simulink library "lib_fuel_converter3"  (Simulink 4.1.1)
values from neighbouring files (symbols this model uses):
  logFlag = 1    [advSACompMaskInit.m]    (also in advSACompMaskInitR13.m)
undefined symbols (not defined in the file or in its folder): air_cp, amb_tmp, cyc_mph, ex_gas_cp, fc_acc_mass, fc_base_mass, fc_c2i_th_cond, fc_c_init_tmp, fc_cl2h_eff, fc_CO2_to_FUELgps, fc_cold, fc_cold_tmp, fc_cp, fc_ct_trq, fc_emisv, fc_ext_sarea, fc_fuel_den, fc_fuel_lhv, fc_h2x_th_cond, fc_h_air_flow, fc_h_cp, fc_h_init_tmp, fc_hood_emisv, fc_hood_sarea, fc_i2x_th_cond, fc_i_init_tmp, fc_inertia, fc_map_spd, fc_map_trq, fc_max_trq, fc_nn_model_name, fc_pwr_scale, fc_spd_scale, fc_trq_scale, fc_tstat, fc_x_init_tmp, fd_ratio, gb_num_init, gb_ratio, generalName, pow, vc_idle_bool, vc_idle_spd, vc_key_on, veh_glider_mass, wh_radius
libraries: lib_fuel_converter3 x4, lib_etc x4, lib_fuel_converter x2, lib_fuel_converter2 x1
(part 2 of 9)

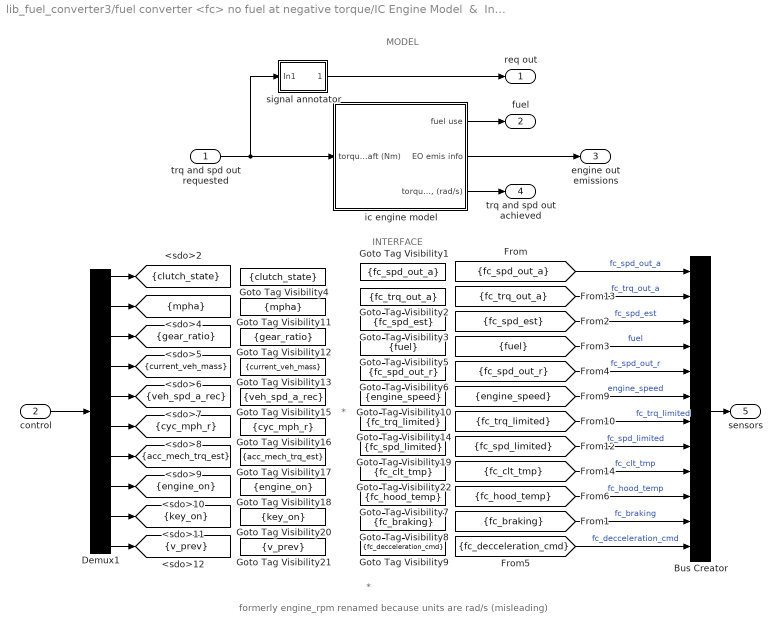
== system lib_fuel_converter3/fuel converter <fc> no fuel at negative torque/IC Engine Model  &  Interface ==
  note: *
  note: *
  note: formerly
      | engine_rpm
      | renamed because
      | units are rad/s
      |  (misleading)
  note: MODEL
  note: INTERFACE
  trq and spd out requested : Inport  Port=1  LatchInput=off
  control : Inport  Port=2  LatchInput=off
  Bus Creator : BusCreator  Inputs=12
  Demux1 : Demux  Outputs=10  BusSelectionMode=off
  Goto Tag Visibility1 : GotoTagVisibility  GotoTag=fc_spd_out_a
  Goto Tag Visibility10 : GotoTagVisibility  GotoTag=engine_speed
  Goto Tag Visibility11 : GotoTagVisibility  GotoTag=mpha
  Goto Tag Visibility12 : GotoTagVisibility  GotoTag=gear_ratio
  Goto Tag Visibility13 : GotoTagVisibility  GotoTag=current_veh_mass
  Goto Tag Visibility14 : GotoTagVisibility  GotoTag=fc_trq_limited
  Goto Tag Visibility15 : GotoTagVisibility  GotoTag=veh_spd_a_rec
  Goto Tag Visibility16 : GotoTagVisibility  GotoTag=cyc_mph_r
  Goto Tag Visibility17 : GotoTagVisibility  GotoTag=acc_mech_trq_est
  Goto Tag Visibility18 : GotoTagVisibility  GotoTag=engine_on
  Goto Tag Visibility19 : GotoTagVisibility  GotoTag=fc_spd_limited
  Goto Tag Visibility2 : GotoTagVisibility  GotoTag=fc_trq_out_a
  Goto Tag Visibility20 : GotoTagVisibility  GotoTag=key_on
  Goto Tag Visibility21 : GotoTagVisibility  GotoTag=v_prev
  Goto Tag Visibility22 : GotoTagVisibility  GotoTag=fc_clt_tmp
  Goto Tag Visibility3 : GotoTagVisibility  GotoTag=fc_spd_est
  Goto Tag Visibility4 : GotoTagVisibility  GotoTag=clutch_state
  Goto Tag Visibility5 : GotoTagVisibility  GotoTag=fuel
  Goto Tag Visibility6 : GotoTagVisibility  GotoTag=fc_spd_out_r
  Goto Tag Visibility7 : GotoTagVisibility  GotoTag=fc_hood_temp
  Goto Tag Visibility8 : GotoTagVisibility  GotoTag=fc_braking
  Goto Tag Visibility9 : GotoTagVisibility  GotoTag=fc_decceleration_cmd
  ic engine model : Subsystem
      settings: RTWFcnNameOpts=Auto  RTWFileNameOpts=Auto
  signal annotator : Subsystem
      settings: RTWFcnNameOpts=Auto  RTWFileNameOpts=Auto
  req out : Outport  Port=1
  fuel : Outport  Port=2
  engine out emissions : Outport  Port=3
  trq and spd out achieved : Outport  Port=4
  sensors : Outport  Port=5
  tag scope: acc_mech_trq_est=scoped, clutch_state=scoped, current_veh_mass=scoped, cyc_mph_r=scoped, engine_on=scoped, gear_ratio=scoped, key_on=scoped, mpha=scoped, v_prev=scoped, veh_spd_a_rec=scoped
  wires:
  [fc_decceleration_cmd] -> Bus Creator/12  "fc_decceleration_cmd"
  Demux1/1 -> [clutch_state]
  Demux1/2 -> [mpha]
  Demux1/3 -> [gear_ratio]
  Demux1/4 -> [current_veh_mass]
  Demux1/5 -> [veh_spd_a_rec]
  Demux1/6 -> [cyc_mph_r]
  Demux1/7 -> [acc_mech_trq_est]
  Demux1/8 -> [engine_on]
  Demux1/9 -> [key_on]
  Demux1/10 -> [v_prev]
  [fc_spd_out_a] -> Bus Creator/1  "fc_spd_out_a"
  [fc_trq_out_a] -> Bus Creator/2  "fc_trq_out_a"
  [fc_spd_est] -> Bus Creator/3  "fc_spd_est"
  [fuel] -> Bus Creator/4  "fuel"
  [fc_spd_out_r] -> Bus Creator/5  "fc_spd_out_r"
  [engine_speed] -> Bus Creator/6  "engine_speed"
  [fc_trq_limited] -> Bus Creator/7  "fc_trq_limited"
  [fc_spd_limited] -> Bus Creator/8  "fc_spd_limited"
  [fc_clt_tmp] -> Bus Creator/9  "fc_clt_tmp"
  [fc_hood_temp] -> Bus Creator/10  "fc_hood_temp"
  trq and spd out requested/1 -> ic engine model/1(torque and speed  req'd at engine  output shaft (Nm)), signal annotator/1(In1)
  ic engine model/1(fuel use) -> fuel/1
  ic engine model/2(EO emis info) -> engine out emissions/1
  ic engine model/3("torque and speed  avail. to driveline (Nm), (rad/s)") -> trq and spd out achieved/1
  control/1 -> Demux1/1
  Bus Creator/1 -> sensors/1
  signal annotator/1(Out1) -> req out/1
  [fc_braking] -> Bus Creator/11  "fc_braking"

== system lib_fuel_converter3/fuel converter <fc> no fuel at negative torque/help ==

== system lib_fuel_converter3/Fuel Converter Control/Fuel Converter Control conventional ic engine/conventional IC engine ==
  note: Controls for Fuel Converter:
      | IC Engine
  Bus Creator : BusCreator  Inputs=10
  Bus Selector1 : BusSelector  OutputSignals=clutch_state  MuxedOutput=off
  Bus Selector2 : BusSelector  OutputSignals=shifting  MuxedOutput=off
  Bus Selector3 : BusSelector  OutputSignals=acc_mech_pwr_a  MuxedOutput=off
  Bus Selector4 : BusSelector  OutputSignals=v_prev  MuxedOutput=off
  Bus Selector5 : BusSelector  OutputSignals=cycle_mph_r  MuxedOutput=off
  Bus Selector6 : BusSelector  OutputSignals=veh_spd_a_rec  MuxedOutput=off
  Bus Selector7 : BusSelector  OutputSignals=gear_ratio  MuxedOutput=off
  Bus Selector8 : BusSelector  OutputSignals=current_veh_mass  MuxedOutput=off
  Bus Selector9 : BusSelector  OutputSignals=mpha  MuxedOutput=off
  Fuel Converter Control : Subsystem
      settings: RTWFcnNameOpts=Auto  RTWFileNameOpts=Auto
  Memory{1..3,5} (4 alike) : Memory  X0=0  InheritSampleTime=off
      settings: RTWStateStorageClass=Auto
  tag scope: fcControl=global
  wires:
  Bus Selector2/1 -> Fuel Converter Control/9(shifting)  "<shifting>"
  Bus Selector7/1 -> Fuel Converter Control/3(gear_ratio)  "<gear_ratio>"
  Bus Selector1/1 -> Fuel Converter Control/1(clutch_state)  "<clutch_state>"
  [clControl] -> Bus Selector1/1
  [gbControl] -> Bus Selector7/1
  [fcSensors] -> Fuel Converter Control/8(fcSensors)
  [vehReqOut] -> Bus Selector4/1
  Bus Selector4/1 -> Fuel Converter Control/10(v_prev)  "<v_prev>"
  [gbControl] -> Bus Selector2/1
  [accSensors] -> Bus Selector3/1
  Bus Selector3/1 -> Memory5/1  "<acc_mech_pwr_a>"
  Memory5/1 -> Fuel Converter Control/7(acc_mech_trq_est)
  [cycReqOut] -> Bus Selector5/1
  Bus Selector5/1 -> Memory3/1  "<cycle_mph_r>"
  [vehSensors] -> Bus Selector6/1
  Bus Selector6/1 -> Memory2/1  "<veh_spd_a_rec>"
  [cycSensors] -> Bus Selector8/1
  Bus Selector8/1 -> Fuel Converter Control/4(current_veh_mass)  "<current_veh_mass>"
  [vehSensors] -> Bus Selector9/1
  Bus Selector9/1 -> Memory1/1  "<mpha>"
  Fuel Converter Control/10(v_prev out) -> Bus Creator/10  "v_prev"
  Fuel Converter Control/9(key_on out) -> Bus Creator/9  "key_on"
  Fuel Converter Control/8(engine_on out) -> Bus Creator/8  "engine_on"
  Fuel Converter Control/7(acc_mech_trq_est out) -> Bus Creator/7  "acc_mech_trq_est"
  Fuel Converter Control/6(cyc_mph_r out) -> Bus Creator/6  "cyc_mph_r_prev"
  Fuel Converter Control/5(veh spd a rec out) -> Bus Creator/5  "veh_spd_a_rec_prev"
  Fuel Converter Control/4(current veh mass out) -> Bus Creator/4  "current_veh_mass"
  Fuel Converter Control/3(gear_ratio out) -> Bus Creator/3  "gear_ratio"
  Fuel Converter Control/2(miles per hour out) -> Bus Creator/2  "mpha_prev"
  Fuel Converter Control/1(clutch state out) -> Bus Creator/1  "clutch_state"
  Bus Creator/1 -> [fcControl]
  Memory1/1 -> Fuel Converter Control/2(mpha(t-1) (prev))
  Memory2/1 -> Fuel Converter Control/5(veh_spd_a_rec(t-1) (prev))
  Memory3/1 -> Fuel Converter Control/6(cyc_mph_r(t-1) (prev))

== system lib_fuel_converter3/configurable subsystems/fuel use and EO emis/Block NOTES ==
  note: This block determines actual fuel use and engine-out emissions
      | given the fully hot values and the engine coolant temperature.
      | The correlations used here were developed at NREL using
      | FTP data collected under subcontract by JDM & Associates.
      | Note: PM hot/cold relation assumed same as HC

== system lib_fuel_converter3/configurable subsystems/fuel use and EO emis/HOT engine maps ==
  T (Nm) : Inport  Port=1  LatchInput=off
  w (rad/s) : Inport  Port=2  LatchInput=off
  Enable : EnablePort  StatesWhenEnabling=reset
  Block NOTES : Subsystem
      settings: RTWFcnNameOpts=Auto  RTWFileNameOpts=Auto
      mask Display: disp('Block\nNOTES')
  CO (g/s) : Subsystem  mask(2-D Table Lookup){@1=fc_map_spd*fc_spd_scale, @2=fc_map_trq*fc_trq_scale, @3=fc_co_map*fc_spd_scale*fc_trq_scale}
      mask prompts: @1 "X Index"; @2 "Y Index"; @3 "Table"
      mask help:
      | Two Dimensional Table Lookup
      | The first input corresponds to X Index and the second input corresponds to the Y Index
      mask init:
      | xindex=@1; yindex=@2; table=@3; sftab2chk(xindex,yindex,table);
      settings: RTWFcnNameOpts=Auto  RTWFileNameOpts=Auto
      mask Help: This block returns a linearly interpolated intersection from the table using the X index (which corresponds to the rows of the table) and the Y index (which corresponds to the columns of the table).  Extrapolation is used.
      mask Display: plot(-10,-10,110,110,[90,50,10],[90,40,30],[90,50,10],[50,26,20],[90,50,10],[22,13,10])
  Fcn3 : Fcn  Expr=(u(1)/1000)*ex_gas_cp*(u(2) - amb_tmp)
  HC (g/s) : Subsystem  mask(2-D Table Lookup){@1=fc_map_spd*fc_spd_scale, @2=fc_map_trq*fc_trq_scale, @3=fc_hc_map*fc_spd_scale*fc_trq_scale}
      mask prompts: @1 "X Index"; @2 "Y Index"; @3 "Table"
      mask help:
      | Two Dimensional Table Lookup
      | The first input corresponds to X Index and the second input corresponds to the Y Index
      mask init:
      | xindex=@1; yindex=@2; table=@3; sftab2chk(xindex,yindex,table);
      settings: RTWFcnNameOpts=Auto  RTWFileNameOpts=Auto
      mask Help: This block returns a linearly interpolated intersection from the table using the X index (which corresponds to the rows of the table) and the Y index (which corresponds to the columns of the table).  Extrapolation is used.
      mask Display: plot(-10,-10,110,110,[90,50,10],[90,40,30],[90,50,10],[50,26,20],[90,50,10],[22,13,10])
  MF,ex (g/s) : Subsystem  mask(2-D Table Lookup){@1=fc_map_spd*fc_spd_scale, @2=fc_map_trq*fc_trq_scale, @3=fc_exflow_map*fc_spd_scale*fc_trq_scale}
      mask prompts: @1 "X Index"; @2 "Y Index"; @3 "Table"
      mask help:
      | Two Dimensional Table Lookup
      | The first input corresponds to X Index and the second input corresponds to the Y Index
      mask init:
      | xindex=@1; yindex=@2; table=@3; sftab2chk(xindex,yindex,table);
      settings: RTWFcnNameOpts=Auto  RTWFileNameOpts=Auto
      mask Help: This block returns a linearly interpolated intersection from the table using the X index (which corresponds to the rows of the table) and the Y index (which corresponds to the columns of the table).  Extrapolation is used.
      mask Display: plot(-10,-10,110,110,[90,50,10],[90,40,30],[90,50,10],[50,26,20],[90,50,10],[22,13,10])
  MinMax : MinMax  Function=min  Inputs=2
  Mux : Mux  Inputs=4
      settings: DisplayOption=none
  Mux4 : Mux  Inputs=2
      settings: DisplayOption=none
  NOx (g/s) : Subsystem  mask(2-D Table Lookup){@1=fc_map_spd*fc_spd_scale, @2=fc_map_trq*fc_trq_scale, @3=fc_nox_map*fc_spd_scale*fc_trq_scale}
      mask prompts: @1 "X Index"; @2 "Y Index"; @3 "Table"
      mask help:
      | Two Dimensional Table Lookup
      | The first input corresponds to X Index and the second input corresponds to the Y Index
      mask init:
      | xindex=@1; yindex=@2; table=@3; sftab2chk(xindex,yindex,table);
      settings: RTWFcnNameOpts=Auto  RTWFileNameOpts=Auto
      mask Help: This block returns a linearly interpolated intersection from the table using the X index (which corresponds to the rows of the table) and the Y index (which corresponds to the columns of the table).  Extrapolation is used.
      mask Display: plot(-10,-10,110,110,[90,50,10],[90,40,30],[90,50,10],[50,26,20],[90,50,10],[22,13,10])
  O2 (g/s) : Subsystem  mask(2-D Table Lookup){@1=fc_map_spd*fc_spd_scale, @2=fc_map_trq*fc_trq_scale, @3=fc_o2_map*fc_spd_scale*fc_trq_scale}
      mask prompts: @1 "X Index"; @2 "Y Index"; @3 "Table"
      mask help:
      | Two Dimensional Table Lookup
      | The first input corresponds to X Index and the second input corresponds to the Y Index
      mask init:
      | xindex=@1; yindex=@2; table=@3; sftab2chk(xindex,yindex,table);
      settings: RTWFcnNameOpts=Auto  RTWFileNameOpts=Auto
      mask Help: This block returns a linearly interpolated intersection from the table using the X index (which corresponds to the rows of the table) and the Y index (which corresponds to the columns of the table).  Extrapolation is used.
      mask Display: plot(-10,-10,110,110,[90,50,10],[90,40,30],[90,50,10],[50,26,20],[90,50,10],[22,13,10])
  PM (g/s) : Subsystem  mask(2-D Table Lookup){@1=fc_map_spd*fc_spd_scale, @2=fc_map_trq*fc_trq_scale, @3=fc_pm_map*fc_spd_scale*fc_trq_scale}
      mask prompts: @1 "X Index"; @2 "Y Index"; @3 "Table"
      mask help:
      | Two Dimensional Table Lookup
      | The first input corresponds to X Index and the second input corresponds to the Y Index
      mask init:
      | xindex=@1; yindex=@2; table=@3; sftab2chk(xindex,yindex,table);
      settings: RTWFcnNameOpts=Auto  RTWFileNameOpts=Auto
      mask Help: This block returns a linearly interpolated intersection from the table using the X index (which corresponds to the rows of the table) and the Y index (which corresponds to the columns of the table).  Extrapolation is used.
      mask Display: plot(-10,-10,110,110,[90,50,10],[90,40,30],[90,50,10],[50,26,20],[90,50,10],[22,13,10])
  Product : Product  Inputs=2  Multiplication=Element-wise(.*)  SaturateOnIntegerOverflow=on
  Saturation : Saturate  UpperLimit=max(fc_map_trq*fc_trq_scale)  LowerLimit=min(fc_map_trq*fc_trq_scale)  LinearizeAsGain=on
  Saturation1 : Saturate  UpperLimit=max(fc_map_spd*fc_spd_scale)  LowerLimit=min(fc_map_spd*fc_spd_scale)  LinearizeAsGain=on
  Sum5 : Sum  Inputs=-+  SaturateOnIntegerOverflow=on
  Sum6 : Sum  Inputs=-+  SaturateOnIntegerOverflow=on
  Tex,eo (C) : Subsystem  mask(2-D Table Lookup){@1=fc_map_spd*fc_spd_scale, @2=fc_map_trq*fc_trq_scale, @3=fc_extmp_map}
      mask prompts: @1 "X Index"; @2 "Y Index"; @3 "Table"
      mask help:
      | Two Dimensional Table Lookup
      | The first input corresponds to X Index and the second input corresponds to the Y Index
      mask init:
      | xindex=@1; yindex=@2; table=@3; sftab2chk(xindex,yindex,table);
      settings: RTWFcnNameOpts=Auto  RTWFileNameOpts=Auto
      mask Help: This block returns a linearly interpolated intersection from the table using the X index (which corresponds to the rows of the table) and the Y index (which corresponds to the columns of the table).  Extrapolation is used.
      mask Display: plot(-10,-10,110,110,[90,50,10],[90,40,30],[90,50,10],[50,26,20],[90,50,10],[22,13,10])
  fuel (g/s) : Subsystem  mask(2-D Table Lookup){@1=fc_map_spd*fc_spd_scale, @2=fc_map_trq*fc_trq_scale, @3=fc_fuel_map*fc_spd_scale*fc_trq_scale}
      mask prompts: @1 "X Index"; @2 "Y Index"; @3 "Table"
      mask help:
      | Two Dimensional Table Lookup
      | The first input corresponds to X Index and the second input corresponds to the Y Index
      mask init:
      | xindex=@1; yindex=@2; table=@3; sftab2chk(xindex,yindex,table);
      settings: RTWFcnNameOpts=Auto  RTWFileNameOpts=Auto
      mask Help: This block returns a linearly interpolated intersection from the table using the X index (which corresponds to the rows of the table) and the Y index (which corresponds to the columns of the table).  Extrapolation is used.
      mask Display: plot(-10,-10,110,110,[90,50,10],[90,40,30],[90,50,10],[50,26,20],[90,50,10],[22,13,10])
  lhv : Gain  Gain=fc_fuel_lhv  Multiplication=Element-wise(K.*u)  SaturateOnIntegerOverflow=on
  fc heat (W) : Outport  Port=1  OutputWhenDisabled=reset  InitialOutput=eps
  HOT fuel use (g/s) : Outport  Port=2  OutputWhenDisabled=reset  InitialOutput=eps
  HOT emis (g/s) : Outport  Port=3  OutputWhenDisabled=reset  InitialOutput=eps
  Ex Gas Flow (g/s) : Outport  Port=4  OutputWhenDisabled=reset  InitialOutput=eps
  Ex Gas Temp (C) : Outport  Port=5  OutputWhenDisabled=reset  InitialOutput=amb_tmp
  O2 exhaust (g/s) : Outport  Port=6  OutputWhenDisabled=reset  InitialOutput=0
  ex heat (W) : Outport  Port=7  OutputWhenDisabled=reset  InitialOutput=eps
  wires:
  PM (g/s)/1(table out) -> Mux/4
  HC (g/s)/1(table out) -> Mux/1
  CO (g/s)/1(table out) -> Mux/2
  NOx (g/s)/1(table out) -> Mux/3
  Mux/1 -> HOT emis (g/s)/1
  MF,ex (g/s)/1(table out) -> Ex Gas Flow (g/s)/1, Mux4/1
  Tex,eo (C)/1(table out) -> Ex Gas Temp (C)/1, Mux4/2
  Saturation1/1 -> NOx (g/s)/1(x0), MF,ex (g/s)/1(x0), Tex,eo (C)/1(x0), fuel (g/s)/1(x0), O2 (g/s)/1(x0), PM (g/s)/1(x0), CO (g/s)/1(x0), HC (g/s)/1(x0)
  Saturation/1 -> CO (g/s)/2(y0), MF,ex (g/s)/2(y0), Tex,eo (C)/2(y0), fuel (g/s)/2(y0), O2 (g/s)/2(y0), PM (g/s)/2(y0), NOx (g/s)/2(y0), HC (g/s)/2(y0)
  T (Nm)/1 -> Saturation/1, Product/1
  w (rad/s)/1 -> Saturation1/1, Product/2
  Mux4/1 -> Fcn3/1
  Sum5/1 -> fc heat (W)/1
  Fcn3/1 -> MinMax/1
  MinMax/1 -> Sum5/1, ex heat (W)/1
  Sum6/1 -> Sum5/2, MinMax/2
  Product/1 -> Sum6/1
  fuel (g/s)/1(table out) -> HOT fuel use (g/s)/1, lhv/1
  lhv/1 -> Sum6/2
  O2 (g/s)/1(table out) -> O2 exhaust (g/s)/1

== system lib_fuel_converter3/configurable subsystems/fuel use and EO emis/enhancedToWorkspace1 ==
  In1 : Inport  Port=1  LatchInput=off
  Terminator : Terminator
  wires:
  In1/1 -> Terminator/1

== system lib_fuel_converter3/configurable subsystems/fuel use and EO emis/enhancedToWorkspace10 ==
  In1 : Inport  Port=1  LatchInput=off
  Terminator : Terminator
  wires:
  In1/1 -> Terminator/1

== system lib_fuel_converter3/configurable subsystems/fuel use and EO emis/enhancedToWorkspace11 ==
  In1 : Inport  Port=1  LatchInput=off
  Terminator : Terminator
  wires:
  In1/1 -> Terminator/1

== system lib_fuel_converter3/configurable subsystems/fuel use and EO emis/enhancedToWorkspace12 ==
  In1 : Inport  Port=1  LatchInput=off
  Terminator : Terminator
  wires:
  In1/1 -> Terminator/1

== system lib_fuel_converter3/configurable subsystems/fuel use and EO emis/enhancedToWorkspace2 ==
  In1 : Inport  Port=1  LatchInput=off
  Terminator : Terminator
  wires:
  In1/1 -> Terminator/1

== system lib_fuel_converter3/configurable subsystems/fuel use and EO emis/enhancedToWorkspace3 ==
  In1 : Inport  Port=1  LatchInput=off
  Terminator : Terminator
  wires:
  In1/1 -> Terminator/1

== system lib_fuel_converter3/configurable subsystems/fuel use and EO emis/enhancedToWorkspace5 ==
  In1 : Inport  Port=1  LatchInput=off
  Terminator : Terminator
  wires:
  In1/1 -> Terminator/1

== system lib_fuel_converter3/configurable subsystems/fuel use and EO emis/enhancedToWorkspace6 ==
  In1 : Inport  Port=1  LatchInput=off
  Terminator : Terminator
  wires:
  In1/1 -> Terminator/1

== system lib_fuel_converter3/configurable subsystems/fuel use and EO emis/enhancedToWorkspace7 ==
  In1 : Inport  Port=1  LatchInput=off
  Terminator : Terminator
  wires:
  In1/1 -> Terminator/1

== system lib_fuel_converter3/configurable subsystems/fuel use and EO emis/enhancedToWorkspace8 ==
  In1 : Inport  Port=1  LatchInput=off
  Terminator : Terminator
  wires:
  In1/1 -> Terminator/1

== system lib_fuel_converter3/configurable subsystems/fuel use and EO emis/enhancedToWorkspace9 ==
  In1 : Inport  Port=1  LatchInput=off
  Terminator : Terminator
  wires:
  In1/1 -> Terminator/1

== system lib_fuel_converter3/configurable subsystems/fuel use and EO emis/fc temp ==
  note: h
  note: x
  note: i
  note: c
  veh spd (m/s) : Inport  Port=1  LatchInput=off
  key ON? : Inport  Orientation=down  Port=2  LatchInput=off
  fc ON? : Inport  Port=3  LatchInput=off
  Qfc (W) : Inport  Port=4  LatchInput=off
  1/ : Gain  Gain=1/(0.2*fc_base_mass*fc_pwr_scale*fc_cp)  Multiplication=Element-wise(K.*u)  SaturateOnIntegerOverflow=on
  1/Ci : Gain  Gain=1/(0.8*fc_base_mass*fc_pwr_scale*fc_cp)  Multiplication=Element-wise(K.*u)  SaturateOnIntegerOverflow=on
  1/Cx : Gain  Gain=1/(fc_acc_mass*fc_pwr_scale*fc_cp)  Multiplication=Element-wise(K.*u)  SaturateOnIntegerOverflow=on
  1/mcp : Gain  Gain=1/(0.1*veh_glider_mass*fc_pwr_scale*fc_h_cp)  Multiplication=Element-wise(K.*u)  SaturateOnIntegerOverflow=on
  Block NOTES : Subsystem
      settings: RTWFcnNameOpts=Auto  RTWFileNameOpts=Auto
      mask Display: disp('Block\nNOTES')
  Memory : Memory  X0=fc_h_init_tmp  InheritSampleTime=off
      settings: RTWStateStorageClass=Auto
  Mux3 : Mux  Inputs=4
      settings: DisplayOption=none
  Mux4 : Mux  Inputs=2
      settings: DisplayOption=none
  Qc : Sum  Inputs=++  SaturateOnIntegerOverflow=on
  Qc1 : Sum  Inputs=--+  SaturateOnIntegerOverflow=on
  Tcm : Integrator  ExternalReset=none  InitialConditionSource=internal  InitialCondition=fc_c_init_tmp  LimitOutput=off  UpperSaturationLimit=inf  LowerSaturationLimit=-inf  ShowSaturationPort=off  ShowStatePort=off  AbsoluteTolerance=auto
  Tcx : Integrator  ExternalReset=none  InitialConditionSource=internal  InitialCondition=fc_x_init_tmp  LimitOutput=off  UpperSaturationLimit=inf  LowerSaturationLimit=-inf  ShowSaturationPort=off  ShowStatePort=off  AbsoluteTolerance=auto
  Tcx1 : Integrator  ExternalReset=none  InitialConditionSource=internal  InitialCondition=fc_i_init_tmp  LimitOutput=off  UpperSaturationLimit=inf  LowerSaturationLimit=-inf  ShowSaturationPort=off  ShowStatePort=off  AbsoluteTolerance=auto
  Tm : Integrator  ExternalReset=none  InitialConditionSource=internal  InitialCondition=fc_h_init_tmp  LimitOutput=off  UpperSaturationLimit=inf  LowerSaturationLimit=-inf  ShowSaturationPort=off  ShowStatePort=off  AbsoluteTolerance=auto
  fc coolant : Subsystem  TreatAsAtomicUnit=on
      settings: RTWFcnNameOpts=Auto  RTWFileNameOpts=Auto
  fc mass heat flow : Subsystem
      settings: RTWFcnNameOpts=Auto  RTWFileNameOpts=Auto
  old fc coolant  temp. (C) : Subsystem
      settings: RTWFcnNameOpts=Auto  RTWFileNameOpts=Auto
  Tfc_old  (C) : Outport  Port=1  InitialOutput=0
  Qfc r,h : Outport  Port=2  InitialOutput=0
  Tfc  (C) : Outport  Port=3  InitialOutput=0
  tag scope: fc_hood_temp=scoped
  wires:
  Qc/1 -> 1//1
  1//1 -> Tcm/1
  Qfc (W)/1 -> Qc/1
  fc mass heat flow/1(Qfc_c) -> Qc/2
  Qc1/1 -> 1/Ci/1
  1/Ci/1 -> Tcx1/1
  Tcm/1 -> Mux3/1
  fc mass heat flow/2(Qfc_i) -> Qc1/3, fc coolant/2("Qfc_i ")
  fc coolant/2(Qfc_htr) -> Qc1/2, Mux4/2
  fc coolant/1(Qfc_rad) -> Qc1/1, Mux4/1
  Tcx1/1 -> fc coolant/1(Tcl), Mux3/2
  Mux4/1 -> Qfc r,h/1
  1/Cx/1 -> Tcx/1
  fc mass heat flow/3(Qfc_x) -> 1/Cx/1
  key ON?/1 -> fc coolant/Enable
  Tcx/1 -> Mux3/3
  Tm/1 -> Mux3/4, Memory/1
  1/mcp/1 -> Tm/1
  fc mass heat flow/4(Qfc_h) -> 1/mcp/1
  Mux3/1 -> fc mass heat flow/2(fc_temp), Tfc  (C)/1
  old fc coolant  temp. (C)/1(fc coolant  temp (C)) -> Tfc_old  (C)/1
  veh spd (m/s)/1 -> old fc coolant  temp. (C)/2(veh spd), fc mass heat flow/1(veh spd)
  fc ON?/1 -> old fc coolant  temp. (C)/1(fc on?)
  Memory/1 -> [fc_hood_temp]

== system lib_fuel_converter3/configurable subsystems/fuel use and EO emis/fc temp correct ==
  Coolant T (C) : Inport  Port=1  LatchInput=off
  HOT fuel use (g/s) : Inport  Port=2  LatchInput=off
  HOT emis (g/s) : Inport  Port=3  LatchInput=off
  T (Nm) : Inport  Port=4  LatchInput=off
  w (rad/s) : Inport  Port=5  LatchInput=off
  Enable : EnablePort  StatesWhenEnabling=reset
  =1: use map based =0: use constant equation based : Constant  Value=fc_cold
  Switch : Switch  Threshold=eps
  Switch1 : Switch  Threshold=eps
  fc temp correct Constant Correction Factors (Equation Based) : Subsystem  TreatAsAtomicUnit=on
      settings: RTWFcnNameOpts=Auto  RTWFileNameOpts=Auto
  fc temp correct Variable Correction Factors (Map Based) : Subsystem  TreatAsAtomicUnit=on
      settings: RTWFcnNameOpts=Auto  RTWFileNameOpts=Auto
  fc_cold=0 : Logic  Operator=NOT  Inputs=2
  fuel use (g/s) : Outport  Port=1  OutputWhenDisabled=reset  InitialOutput=0
  EO emis (g/s) : Outport  Port=2  OutputWhenDisabled=reset  InitialOutput=0
  wires:
  =1: use map based =0: use constant equation based/1 -> fc_cold=0/1, fc temp correct Variable Correction Factors (Map Based)/Enable
  Coolant T (C)/1 -> fc temp correct Constant Correction Factors (Equation Based)/1(Coolant T (C)), fc temp correct Variable Correction Factors (Map Based)/1(Coolant T (C))
  HOT fuel use (g/s)/1 -> fc temp correct Constant Correction Factors (Equation Based)/2(HOT fuel use (g/s)), fc temp correct Variable Correction Factors (Map Based)/2(HOT fuel use (g/s))
  HOT emis (g/s)/1 -> fc temp correct Constant Correction Factors (Equation Based)/3(HOT emis (g/s)), fc temp correct Variable Correction Factors (Map Based)/3(HOT emis (g/s))
  fc temp correct Constant Correction Factors (Equation Based)/1(fuel use (g/s)) -> Switch/1
  fc_cold=0/1 -> fc temp correct Constant Correction Factors (Equation Based)/Enable, Switch/2, Switch1/2
  fc temp correct Variable Correction Factors (Map Based)/1(fuel use (g/s)) -> Switch/3
  fc temp correct Constant Correction Factors (Equation Based)/2(EO emis (g/s)) -> Switch1/1
  fc temp correct Variable Correction Factors (Map Based)/2(EO emis (g/s)) -> Switch1/3
  Switch/1 -> fuel use (g/s)/1
  Switch1/1 -> EO emis (g/s)/1
  T (Nm)/1 -> fc temp correct Variable Correction Factors (Map Based)/4(T (Nm))
  w (rad/s)/1 -> fc temp correct Variable Correction Factors (Map Based)/5(w (rad/s))

== system lib_fuel_converter3/configurable subsystems/fuel use and EO emis Neural Network Model/HOT engine maps ==
  T (Nm) : Inport  Port=1  LatchInput=off
  w (rad/s) : Inport  Port=2  LatchInput=off
  Enable : EnablePort  StatesWhenEnabling=reset
  Block NOTES : Subsystem
      settings: RTWFcnNameOpts=Auto  RTWFileNameOpts=Auto
      mask Display: disp('Block\nNOTES')
  CO (g/s) : Subsystem  mask(2-D Table Lookup){@1=fc_map_spd*fc_spd_scale, @2=fc_map_trq*fc_trq_scale, @3=fc_co_map*fc_spd_scale*fc_trq_scale}
      mask prompts: @1 "X Index"; @2 "Y Index"; @3 "Table"
      mask help:
      | Two Dimensional Table Lookup
      | The first input corresponds to X Index and the second input corresponds to the Y Index
      mask init:
      | xindex=@1; yindex=@2; table=@3; sftab2chk(xindex,yindex,table);
      settings: RTWFcnNameOpts=Auto  RTWFileNameOpts=Auto
      mask Help: This block returns a linearly interpolated intersection from the table using the X index (which corresponds to the rows of the table) and the Y index (which corresponds to the columns of the table).  Extrapolation is used.
      mask Display: plot(-10,-10,110,110,[90,50,10],[90,40,30],[90,50,10],[50,26,20],[90,50,10],[22,13,10])
  Fcn3 : Fcn  Expr=(u(1)/1000)*ex_gas_cp*(u(2) - amb_tmp)
  HC (g/s) : Subsystem  mask(2-D Table Lookup){@1=fc_map_spd*fc_spd_scale, @2=fc_map_trq*fc_trq_scale, @3=fc_hc_map*fc_spd_scale*fc_trq_scale}
      mask prompts: @1 "X Index"; @2 "Y Index"; @3 "Table"
      mask help:
      | Two Dimensional Table Lookup
      | The first input corresponds to X Index and the second input corresponds to the Y Index
      mask init:
      | xindex=@1; yindex=@2; table=@3; sftab2chk(xindex,yindex,table);
      settings: RTWFcnNameOpts=Auto  RTWFileNameOpts=Auto
      mask Help: This block returns a linearly interpolated intersection from the table using the X index (which corresponds to the rows of the table) and the Y index (which corresponds to the columns of the table).  Extrapolation is used.
      mask Display: plot(-10,-10,110,110,[90,50,10],[90,40,30],[90,50,10],[50,26,20],[90,50,10],[22,13,10])
  MF,ex (g/s) : Subsystem  mask(2-D Table Lookup){@1=fc_map_spd*fc_spd_scale, @2=fc_map_trq*fc_trq_scale, @3=fc_exflow_map*fc_spd_scale*fc_trq_scale}
      mask prompts: @1 "X Index"; @2 "Y Index"; @3 "Table"
      mask help:
      | Two Dimensional Table Lookup
      | The first input corresponds to X Index and the second input corresponds to the Y Index
      mask init:
      | xindex=@1; yindex=@2; table=@3; sftab2chk(xindex,yindex,table);
      settings: RTWFcnNameOpts=Auto  RTWFileNameOpts=Auto
      mask Help: This block returns a linearly interpolated intersection from the table using the X index (which corresponds to the rows of the table) and the Y index (which corresponds to the columns of the table).  Extrapolation is used.
      mask Display: plot(-10,-10,110,110,[90,50,10],[90,40,30],[90,50,10],[50,26,20],[90,50,10],[22,13,10])
  MinMax : MinMax  Function=min  Inputs=2
  Mux : Mux  Inputs=4
      settings: DisplayOption=none
  Mux4 : Mux  Inputs=2
      settings: DisplayOption=none
  NOx (g/s) : Subsystem  mask(2-D Table Lookup){@1=fc_map_spd*fc_spd_scale, @2=fc_map_trq*fc_trq_scale, @3=fc_nox_map*fc_spd_scale*fc_trq_scale}
      mask prompts: @1 "X Index"; @2 "Y Index"; @3 "Table"
      mask help:
      | Two Dimensional Table Lookup
      | The first input corresponds to X Index and the second input corresponds to the Y Index
      mask init:
      | xindex=@1; yindex=@2; table=@3; sftab2chk(xindex,yindex,table);
      settings: RTWFcnNameOpts=Auto  RTWFileNameOpts=Auto
      mask Help: This block returns a linearly interpolated intersection from the table using the X index (which corresponds to the rows of the table) and the Y index (which corresponds to the columns of the table).  Extrapolation is used.
      mask Display: plot(-10,-10,110,110,[90,50,10],[90,40,30],[90,50,10],[50,26,20],[90,50,10],[22,13,10])
  O2 (g/s) : Subsystem  mask(2-D Table Lookup){@1=fc_map_spd*fc_spd_scale, @2=fc_map_trq*fc_trq_scale, @3=fc_o2_map*fc_spd_scale*fc_trq_scale}
      mask prompts: @1 "X Index"; @2 "Y Index"; @3 "Table"
      mask help:
      | Two Dimensional Table Lookup
      | The first input corresponds to X Index and the second input corresponds to the Y Index
      mask init:
      | xindex=@1; yindex=@2; table=@3; sftab2chk(xindex,yindex,table);
      settings: RTWFcnNameOpts=Auto  RTWFileNameOpts=Auto
      mask Help: This block returns a linearly interpolated intersection from the table using the X index (which corresponds to the rows of the table) and the Y index (which corresponds to the columns of the table).  Extrapolation is used.
      mask Display: plot(-10,-10,110,110,[90,50,10],[90,40,30],[90,50,10],[50,26,20],[90,50,10],[22,13,10])
  PM (g/s) : Subsystem  mask(2-D Table Lookup){@1=fc_map_spd*fc_spd_scale, @2=fc_map_trq*fc_trq_scale, @3=fc_pm_map*fc_spd_scale*fc_trq_scale}
      mask prompts: @1 "X Index"; @2 "Y Index"; @3 "Table"
      mask help:
      | Two Dimensional Table Lookup
      | The first input corresponds to X Index and the second input corresponds to the Y Index
      mask init:
      | xindex=@1; yindex=@2; table=@3; sftab2chk(xindex,yindex,table);
      settings: RTWFcnNameOpts=Auto  RTWFileNameOpts=Auto
      mask Help: This block returns a linearly interpolated intersection from the table using the X index (which corresponds to the rows of the table) and the Y index (which corresponds to the columns of the table).  Extrapolation is used.
      mask Display: plot(-10,-10,110,110,[90,50,10],[90,40,30],[90,50,10],[50,26,20],[90,50,10],[22,13,10])
  Product : Product  Inputs=2  Multiplication=Element-wise(.*)  SaturateOnIntegerOverflow=on
  Saturation : Saturate  UpperLimit=max(fc_map_trq*fc_trq_scale)  LowerLimit=min(fc_map_trq*fc_trq_scale)  LinearizeAsGain=on
  Saturation1 : Saturate  UpperLimit=max(fc_map_spd*fc_spd_scale)  LowerLimit=min(fc_map_spd*fc_spd_scale)  LinearizeAsGain=on
  Sum5 : Sum  Inputs=-+  SaturateOnIntegerOverflow=on
  Sum6 : Sum  Inputs=-+  SaturateOnIntegerOverflow=on
  Tex,eo (C) : Subsystem  mask(2-D Table Lookup){@1=fc_map_spd*fc_spd_scale, @2=fc_map_trq*fc_trq_scale, @3=fc_extmp_map}
      mask prompts: @1 "X Index"; @2 "Y Index"; @3 "Table"
      mask help:
      | Two Dimensional Table Lookup
      | The first input corresponds to X Index and the second input corresponds to the Y Index
      mask init:
      | xindex=@1; yindex=@2; table=@3; sftab2chk(xindex,yindex,table);
      settings: RTWFcnNameOpts=Auto  RTWFileNameOpts=Auto
      mask Help: This block returns a linearly interpolated intersection from the table using the X index (which corresponds to the rows of the table) and the Y index (which corresponds to the columns of the table).  Extrapolation is used.
      mask Display: plot(-10,-10,110,110,[90,50,10],[90,40,30],[90,50,10],[50,26,20],[90,50,10],[22,13,10])
  fuel (g/s) : Subsystem  mask(2-D Table Lookup){@1=fc_map_spd*fc_spd_scale, @2=fc_map_trq*fc_trq_scale, @3=fc_fuel_map*fc_spd_scale*fc_trq_scale}
      mask prompts: @1 "X Index"; @2 "Y Index"; @3 "Table"
      mask help:
      | Two Dimensional Table Lookup
      | The first input corresponds to X Index and the second input corresponds to the Y Index
      mask init:
      | xindex=@1; yindex=@2; table=@3; sftab2chk(xindex,yindex,table);
      settings: RTWFcnNameOpts=Auto  RTWFileNameOpts=Auto
      mask Help: This block returns a linearly interpolated intersection from the table using the X index (which corresponds to the rows of the table) and the Y index (which corresponds to the columns of the table).  Extrapolation is used.
      mask Display: plot(-10,-10,110,110,[90,50,10],[90,40,30],[90,50,10],[50,26,20],[90,50,10],[22,13,10])
  lhv : Gain  Gain=fc_fuel_lhv  Multiplication=Element-wise(K.*u)  SaturateOnIntegerOverflow=on
  fc heat (W) : Outport  Port=1  OutputWhenDisabled=reset  InitialOutput=eps
  HOT fuel use (g/s) : Outport  Port=2  OutputWhenDisabled=reset  InitialOutput=eps
  HOT emis (g/s) : Outport  Port=3  OutputWhenDisabled=reset  InitialOutput=eps
  Ex Gas Flow (g/s) : Outport  Port=4  OutputWhenDisabled=reset  InitialOutput=eps
  Ex Gas Temp (C) : Outport  Port=5  OutputWhenDisabled=reset  InitialOutput=amb_tmp
  O2 exhaust (g/s) : Outport  Port=6  OutputWhenDisabled=reset  InitialOutput=0
  ex heat (W) : Outport  Port=7  OutputWhenDisabled=reset  InitialOutput=eps
  wires:
  PM (g/s)/1(table out) -> Mux/4
  HC (g/s)/1(table out) -> Mux/1
  CO (g/s)/1(table out) -> Mux/2
  NOx (g/s)/1(table out) -> Mux/3
  Mux/1 -> HOT emis (g/s)/1
  MF,ex (g/s)/1(table out) -> Ex Gas Flow (g/s)/1, Mux4/1
  Tex,eo (C)/1(table out) -> Ex Gas Temp (C)/1, Mux4/2
  Saturation1/1 -> NOx (g/s)/1(x0), MF,ex (g/s)/1(x0), Tex,eo (C)/1(x0), fuel (g/s)/1(x0), O2 (g/s)/1(x0), PM (g/s)/1(x0), CO (g/s)/1(x0), HC (g/s)/1(x0)
  Saturation/1 -> CO (g/s)/2(y0), MF,ex (g/s)/2(y0), Tex,eo (C)/2(y0), fuel (g/s)/2(y0), O2 (g/s)/2(y0), PM (g/s)/2(y0), NOx (g/s)/2(y0), HC (g/s)/2(y0)
  T (Nm)/1 -> Saturation/1, Product/1
  w (rad/s)/1 -> Saturation1/1, Product/2
  Mux4/1 -> Fcn3/1
  Sum5/1 -> fc heat (W)/1
  Fcn3/1 -> MinMax/1
  MinMax/1 -> Sum5/1, ex heat (W)/1
  Sum6/1 -> Sum5/2, MinMax/2
  Product/1 -> Sum6/1
  fuel (g/s)/1(table out) -> HOT fuel use (g/s)/1, lhv/1
  lhv/1 -> Sum6/2
  O2 (g/s)/1(table out) -> O2 exhaust (g/s)/1

== system lib_fuel_converter3/configurable subsystems/fuel use and EO emis Neural Network Model/enhancedToWorkspace1 ==
  In1 : Inport  Port=1  LatchInput=off
  Terminator : Terminator
  wires:
  In1/1 -> Terminator/1

== system lib_fuel_converter3/configurable subsystems/fuel use and EO emis Neural Network Model/enhancedToWorkspace12 ==
  In1 : Inport  Port=1  LatchInput=off
  Terminator : Terminator
  wires:
  In1/1 -> Terminator/1

== system lib_fuel_converter3/configurable subsystems/fuel use and EO emis Neural Network Model/enhancedToWorkspace13 ==
  In1 : Inport  Port=1  LatchInput=off
  Terminator : Terminator
  wires:
  In1/1 -> Terminator/1

== system lib_fuel_converter3/configurable subsystems/fuel use and EO emis Neural Network Model/enhancedToWorkspace14 ==
  In1 : Inport  Port=1  LatchInput=off
  Terminator : Terminator
  wires:
  In1/1 -> Terminator/1

== system lib_fuel_converter3/configurable subsystems/fuel use and EO emis Neural Network Model/enhancedToWorkspace15 ==
  In1 : Inport  Port=1  LatchInput=off
  Terminator : Terminator
  wires:
  In1/1 -> Terminator/1

== system lib_fuel_converter3/configurable subsystems/fuel use and EO emis Neural Network Model/enhancedToWorkspace16 ==
  In1 : Inport  Port=1  LatchInput=off
  Terminator : Terminator
  wires:
  In1/1 -> Terminator/1

== system lib_fuel_converter3/configurable subsystems/fuel use and EO emis Neural Network Model/enhancedToWorkspace17 ==
  In1 : Inport  Port=1  LatchInput=off
  Terminator : Terminator
  wires:
  In1/1 -> Terminator/1

== system lib_fuel_converter3/configurable subsystems/fuel use and EO emis Neural Network Model/enhancedToWorkspace18 ==
  In1 : Inport  Port=1  LatchInput=off
  Terminator : Terminator
  wires:
  In1/1 -> Terminator/1

== system lib_fuel_converter3/configurable subsystems/fuel use and EO emis Neural Network Model/enhancedToWorkspace2 ==
  In1 : Inport  Port=1  LatchInput=off
  Terminator : Terminator
  wires:
  In1/1 -> Terminator/1

== system lib_fuel_converter3/configurable subsystems/fuel use and EO emis Neural Network Model/enhancedToWorkspace3 ==
  In1 : Inport  Port=1  LatchInput=off
  Terminator : Terminator
  wires:
  In1/1 -> Terminator/1

== system lib_fuel_converter3/configurable subsystems/fuel use and EO emis Neural Network Model/enhancedToWorkspace5 ==
  In1 : Inport  Port=1  LatchInput=off
  Terminator : Terminator
  wires:
  In1/1 -> Terminator/1

== system lib_fuel_converter3/configurable subsystems/fuel use and EO emis Neural Network Model/enhancedToWorkspace6 ==
  In1 : Inport  Port=1  LatchInput=off
  Terminator : Terminator
  wires:
  In1/1 -> Terminator/1

== system lib_fuel_converter3/configurable subsystems/fuel use and EO emis Neural Network Model/enhancedToWorkspace7 ==
  In1 : Inport  Port=1  LatchInput=off
  Terminator : Terminator
  wires:
  In1/1 -> Terminator/1

== system lib_fuel_converter3/configurable subsystems/fuel use and EO emis Neural Network Model/enhancedToWorkspace8 ==
  In1 : Inport  Port=1  LatchInput=off
  Terminator : Terminator
  wires:
  In1/1 -> Terminator/1

== system lib_fuel_converter3/configurable subsystems/fuel use and EO emis Neural Network Model/enhancedToWorkspace9 ==
  In1 : Inport  Port=1  LatchInput=off
  Terminator : Terminator
  wires:
  In1/1 -> Terminator/1

== system lib_fuel_converter3/configurable subsystems/fuel use and EO emis Neural Network Model/fc temp ==
  note: c
  note: i
  note: x
  note: h
  veh spd (m/s) : Inport  Port=1  LatchInput=off
  key ON? : Inport  Orientation=down  Port=2  LatchInput=off
  fc ON? : Inport  Port=3  LatchInput=off
  Qfc (W) : Inport  Port=4  LatchInput=off
  1/ : Gain  Gain=1/(0.2*fc_base_mass*fc_pwr_scale*fc_cp)  Multiplication=Element-wise(K.*u)  SaturateOnIntegerOverflow=on
  1/Ci : Gain  Gain=1/(0.8*fc_base_mass*fc_pwr_scale*fc_cp)  Multiplication=Element-wise(K.*u)  SaturateOnIntegerOverflow=on
  1/Cx : Gain  Gain=1/(fc_acc_mass*fc_pwr_scale*fc_cp)  Multiplication=Element-wise(K.*u)  SaturateOnIntegerOverflow=on
  1/mcp : Gain  Gain=1/(0.1*veh_glider_mass*fc_pwr_scale*fc_h_cp)  Multiplication=Element-wise(K.*u)  SaturateOnIntegerOverflow=on
  Block NOTES : Subsystem
      settings: RTWFcnNameOpts=Auto  RTWFileNameOpts=Auto
      mask Display: disp('Block\nNOTES')
  Memory : Memory  X0=fc_h_init_tmp  InheritSampleTime=off
      settings: RTWStateStorageClass=Auto
  Mux3 : Mux  Inputs=4
      settings: DisplayOption=none
  Mux4 : Mux  Inputs=2
      settings: DisplayOption=none
  Qc : Sum  Inputs=++  SaturateOnIntegerOverflow=on
  Qc1 : Sum  Inputs=--+  SaturateOnIntegerOverflow=on
  Tcm : Integrator  ExternalReset=none  InitialConditionSource=internal  InitialCondition=fc_c_init_tmp  LimitOutput=off  UpperSaturationLimit=inf  LowerSaturationLimit=-inf  ShowSaturationPort=off  ShowStatePort=off  AbsoluteTolerance=auto
  Tcx : Integrator  ExternalReset=none  InitialConditionSource=internal  InitialCondition=fc_x_init_tmp  LimitOutput=off  UpperSaturationLimit=inf  LowerSaturationLimit=-inf  ShowSaturationPort=off  ShowStatePort=off  AbsoluteTolerance=auto
  Tcx1 : Integrator  ExternalReset=none  InitialConditionSource=internal  InitialCondition=fc_i_init_tmp  LimitOutput=off  UpperSaturationLimit=inf  LowerSaturationLimit=-inf  ShowSaturationPort=off  ShowStatePort=off  AbsoluteTolerance=auto
  Tm : Integrator  ExternalReset=none  InitialConditionSource=internal  InitialCondition=fc_h_init_tmp  LimitOutput=off  UpperSaturationLimit=inf  LowerSaturationLimit=-inf  ShowSaturationPort=off  ShowStatePort=off  AbsoluteTolerance=auto
  fc coolant : lib_fuel_converter2/configurable subsystems/fuel use and EO emis Neural Network Model/fc temp/fc coolant  TreatAsAtomicUnit=on
      settings: RTWFcnNameOpts=Auto  RTWFileNameOpts=Auto
  fc mass heat flow : Subsystem
      settings: RTWFcnNameOpts=Auto  RTWFileNameOpts=Auto
  old fc coolant  temp. (C) : Subsystem
      settings: RTWFcnNameOpts=Auto  RTWFileNameOpts=Auto
  Tfc_old  (C) : Outport  Port=1  InitialOutput=0
  Qfc r,h : Outport  Port=2  InitialOutput=0
  Tfc  (C) : Outport  Port=3  InitialOutput=0
  tag scope: fc_hood_temp=scoped
  wires:
  fc ON?/1 -> old fc coolant  temp. (C)/1(fc on?)
  veh spd (m/s)/1 -> fc mass heat flow/1(veh spd), old fc coolant  temp. (C)/2(veh spd)
  old fc coolant  temp. (C)/1(fc coolant  temp (C)) -> Tfc_old  (C)/1
  Mux3/1 -> Tfc  (C)/1, fc mass heat flow/2(fc_temp)
  fc mass heat flow/4(Qfc_h) -> 1/mcp/1
  1/mcp/1 -> Tm/1
  Tm/1 -> Mux3/4, Memory/1
  Tcx/1 -> Mux3/3
  key ON?/1 -> fc coolant/Enable
  fc mass heat flow/3(Qfc_x) -> 1/Cx/1
  1/Cx/1 -> Tcx/1
  Mux4/1 -> Qfc r,h/1
  Tcx1/1 -> Mux3/2, fc coolant/1
  fc coolant/1 -> Mux4/1, Qc1/1
  fc coolant/2 -> Mux4/2, Qc1/2
  fc mass heat flow/2(Qfc_i) -> fc coolant/2, Qc1/3
  Tcm/1 -> Mux3/1
  1/Ci/1 -> Tcx1/1
  Qc1/1 -> 1/Ci/1
  fc mass heat flow/1(Qfc_c) -> Qc/2
  Qfc (W)/1 -> Qc/1
  1//1 -> Tcm/1
  Qc/1 -> 1//1
  Memory/1 -> [fc_hood_temp]

== system lib_fuel_converter3/configurable subsystems/fuel use and EO emis Neural Network Model/fc temp correct ==
  Coolant T (C) : Inport  Port=1  LatchInput=off
  HOT fuel use (g/s) : Inport  Port=2  LatchInput=off
  HOT emis (g/s) : Inport  Port=3  LatchInput=off
  T (Nm) : Inport  Port=4  LatchInput=off
  w (rad/s) : Inport  Port=5  LatchInput=off
  Enable : EnablePort  StatesWhenEnabling=reset
  =1: use map based =0: use constant equation based : Constant  Value=fc_cold
  Switch : Switch  Threshold=eps
  Switch1 : Switch  Threshold=eps
  fc temp correct Constant Correction Factors (Equation Based) : Subsystem  TreatAsAtomicUnit=on
      settings: RTWFcnNameOpts=Auto  RTWFileNameOpts=Auto
  fc temp correct Variable Correction Factors (Map Based) : Subsystem  TreatAsAtomicUnit=on
      settings: RTWFcnNameOpts=Auto  RTWFileNameOpts=Auto
  fc_cold=0 : Logic  Operator=NOT  Inputs=2
  fuel use (g/s) : Outport  Port=1  OutputWhenDisabled=reset  InitialOutput=0
  EO emis (g/s) : Outport  Port=2  OutputWhenDisabled=reset  InitialOutput=0
  wires:
  w (rad/s)/1 -> fc temp correct Variable Correction Factors (Map Based)/5(w (rad/s))
  T (Nm)/1 -> fc temp correct Variable Correction Factors (Map Based)/4(T (Nm))
  Switch1/1 -> EO emis (g/s)/1
  Switch/1 -> fuel use (g/s)/1
  fc temp correct Variable Correction Factors (Map Based)/2(EO emis (g/s)) -> Switch1/3
  fc temp correct Constant Correction Factors (Equation Based)/2(EO emis (g/s)) -> Switch1/1
  fc temp correct Variable Correction Factors (Map Based)/1(fuel use (g/s)) -> Switch/3
  fc_cold=0/1 -> Switch1/2, Switch/2, fc temp correct Constant Correction Factors (Equation Based)/Enable
  fc temp correct Constant Correction Factors (Equation Based)/1(fuel use (g/s)) -> Switch/1
  HOT emis (g/s)/1 -> fc temp correct Variable Correction Factors (Map Based)/3(HOT emis (g/s)), fc temp correct Constant Correction Factors (Equation Based)/3(HOT emis (g/s))
  HOT fuel use (g/s)/1 -> fc temp correct Variable Correction Factors (Map Based)/2(HOT fuel use (g/s)), fc temp correct Constant Correction Factors (Equation Based)/2(HOT fuel use (g/s))
  Coolant T (C)/1 -> fc temp correct Variable Correction Factors (Map Based)/1(Coolant T (C)), fc temp correct Constant Correction Factors (Equation Based)/1(Coolant T (C))
  =1: use map based =0: use constant equation based/1 -> fc temp correct Variable Correction Factors (Map Based)/Enable, fc_cold=0/1

== system lib_fuel_converter3/configurable subsystems/fuel use and EO emis Neural Network Model/nn thermal calcs ==
  gpsCO2 : Inport  Port=1  LatchInput=off
  pwr (W) : Inport  Port=2  LatchInput=off
  ex gas flow (g/s) : Inport  Port=3  LatchInput=off
  ex gas tmp : Inport  Port=4  LatchInput=off
  (g/s CO2) to (g/s fuel) : Gain  Gain=fc_CO2_to_FUELgps  Multiplication=Element-wise(K.*u)  SaturateOnIntegerOverflow=on
  Fcn3 : Fcn  Expr=(u(1)/1000)*ex_gas_cp*(u(2) - amb_tmp)
  MinMax : MinMax  Function=min  Inputs=2
  Mux4 : Mux  Inputs=2
      settings: DisplayOption=none
  Sum5 : Sum  Inputs=-+  SaturateOnIntegerOverflow=on
  Sum6 : Sum  Inputs=-+  SaturateOnIntegerOverflow=on
  lhv : Gain  Gain=fc_fuel_lhv  Multiplication=Element-wise(K.*u)  SaturateOnIntegerOverflow=on
  fc heat (W) : Outport  Port=1  OutputWhenDisabled=reset  InitialOutput=eps
  HOT fuel use (g/s) : Outport  Port=2  OutputWhenDisabled=reset  InitialOutput=eps
  ex heat (W) : Outport  Port=3  OutputWhenDisabled=reset  InitialOutput=eps
  wires:
  lhv/1 -> Sum6/2
  [fuel_gps] -> lhv/1, HOT fuel use (g/s)/1
  Sum6/1 -> MinMax/2, Sum5/2
  MinMax/1 -> ex heat (W)/1, Sum5/1
  Fcn3/1 -> MinMax/1
  Sum5/1 -> fc heat (W)/1
  Mux4/1 -> Fcn3/1
  gpsCO2/1 -> (g/s CO2) to (g/s fuel)/1
  (g/s CO2) to (g/s fuel)/1 -> [fuel_gps]
  pwr (W)/1 -> Sum6/1
  ex gas tmp/1 -> Mux4/2
  ex gas flow (g/s)/1 -> Mux4/1
